simulink model "vel"  (R2022a)
settings: Solver=FixedStepAuto  StartTime=0.0  StopTime=2  FixedStep=1e-3  RelTol=1e-3
undefined symbols (not defined in the file or in its folder): phi, r, theta
libraries: robotlib x12, simulink_extras x8, robotgazebolib x4, slpidlib x1, simulink x1
settings Model: Creator=abiyyumufti  LastModifiedBy=abiyyumufti

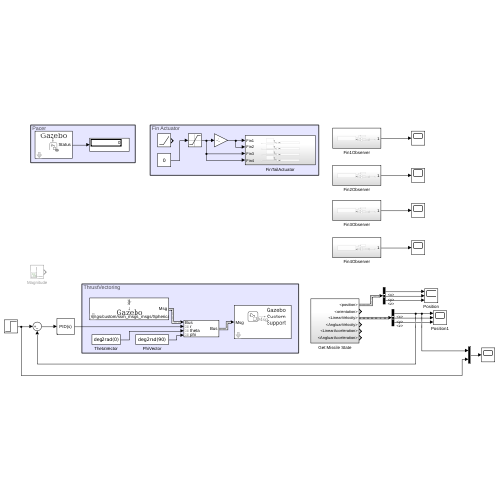
[thumbnail: Simulink's stored preview of the top-level diagram]
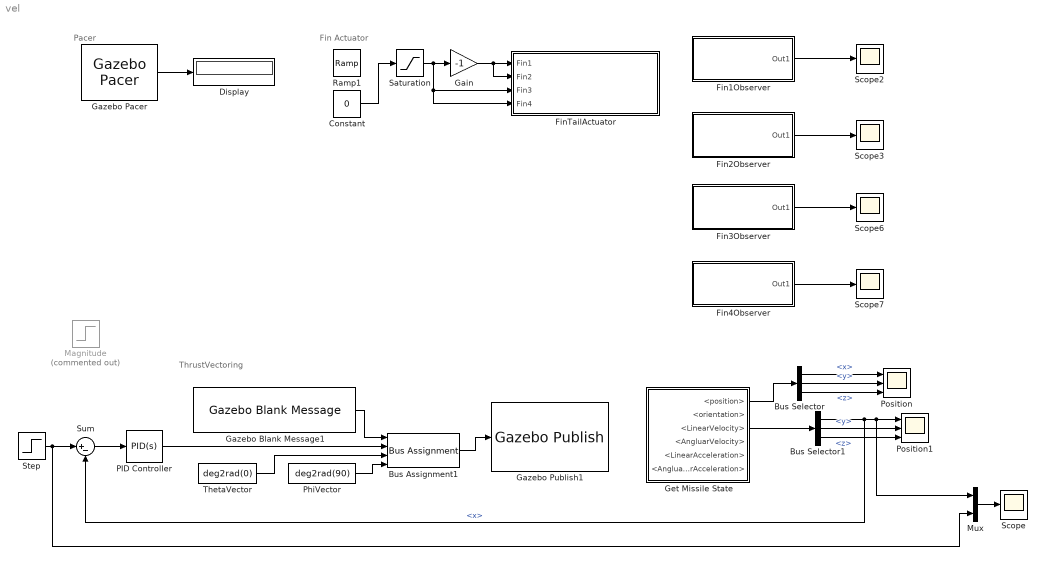
== system vel ==
  note: Fin Actuator
  note: Pacer
  note: ThrustVectoring
  Bus Assignment1 : BusAssignment  AssignedSignals=r,theta,phi
  Bus Selector : BusSelector  OutputSignals=x,y,z
  Bus Selector1 : BusSelector  OutputSignals=x,y,z
  Constant : Constant  Value=0
  Display : Display
  Fin1Observer : Subsystem
  Fin2Observer : Subsystem
  Fin3Observer : Subsystem
  Fin4Observer : Subsystem
  FinTailActuator : Subsystem
  Gain : Gain  Gain=-1
  Gazebo Blank Message1 : robotgazebolib/Gazebo Blank Message  msgType=gazebo_msgs/custom/ssm_msgs_msgs/SphericalVector  sampleTime=0.001  busName='Gazebo_SL_Bus_gazebo_msgs_custom_ssm_msgs_msgs_SphericalVector'
      settings: SourceProductBaseCode=RO
  Gazebo Pacer : robotgazebolib/Gazebo Pacer  ResetBehavior=Reset Gazebo simulation time and scene  SampleTime=0.001
      settings: SourceProductBaseCode=RO
  Gazebo Publish1 : robotgazebolib/Gazebo Publish  topicSource=Specify your own  topic=/gazebo/my_world/thrust_force  messageType=gazebo_msgs/custom/ssm_msgs_msgs/SphericalVector  sampleTime=0.001
      settings: SourceProductBaseCode=RO
  Get Missile State : Subsystem
  Magnitude : Step  Commented=on  Time=2  Before=80000  After=0  SampleTime=0
  Mux : Mux  Inputs=2
  PID Controller : slpidlib/PID Controller  Controller=PID  Form=Parallel  TimeDomain=Continuous-time  UseExternalTs=off  SampleTime=-1  IntegratorMethod=Forward Euler  FilterMethod=Forward Euler  ControllerParametersSource=internal  P=10000  I=0  UseKiTs=off  D=15  N=100  UseFilter=on  TunerSelectOption=Transfer Function Based (PID Tuner App)  InitialConditionSource=internal  InitialConditionForIntegrator=0  InitialConditionForFilter=0  DifferentiatorICPrevScaledInput=0  ExternalReset=none  TrackingMode=off  Kt=1  LimitOutput=off  SatLimitsSource=internal  UpperSaturationLimit=inf  LowerSaturationLimit=-inf  LinearizeAsGain=on  AntiWindupMode=none  Kb=1  POutMin=[]  POutMax=[]  IOutMin=[]  IOutMax=[]  DOutMin=[]  DOutMax=[]  NOutMin=[]  NOutMax=[]  SumOutMin=[]  SumOutMax=[]  SaturationOutMin=[]  SaturationOutMax=[]  PParamMin=[]  PParamMax=[]  IParamMin=[]  IParamMax=[]  DParamMin=[]  DParamMax=[]  NParamMin=[]  NParamMax=[]  KbParamMin=[]  KbParamMax=[]  KtParamMin=[]  KtParamMax=[]  KbOutMin=[]  KbOutMax=[]  KtOutMin=[]  KtOutMax=[]  IntegratorOutMin=[]  IntegratorOutMax=[]  FilterOutMin=[]  FilterOutMax=[]  SumI1OutMin=[]  SumI1OutMax=[]  SumI2OutMin=[]  SumI2OutMax=[]  SumI3OutMin=[]  SumI3OutMax=[]  SumI4OutMin=[]  SumI4OutMax=[]  SumDOutMin=[]  SumDOutMax=[]  DifferentiatorOutMin=[]  DifferentiatorOutMax=[]  FilterDiffOutCoefMin=[]  FilterDiffOutCoefMax=[]  ReciprocalOutMin=[]  ReciprocalOutMax=[]  SumDenOutMin=[]  SumDenOutMax=[]  SumNumOutMin=[]  SumNumOutMax=[]  DivideOutMin=[]  DivideOutMax=[]  UdiffTsProdOutMin=[]  UdiffTsProdOutMax=[]  NTsProdOutMin=[]  NTsProdOutMax=[]  UintegralTsProdOutMin=[]  UintegralTsProdOutMax=[]  UngainTsProdOutMin=[]  UngainTsProdOutMax=[]  IntegratorContinuousStateAttributes=''  IntegratorStateMustResolveToSignalObject=off  IntegratorRTWStateStorageClass=Auto  FilterContinuousStateAttributes=''  FilterStateMustResolveToSignalObject=off  FilterRTWStateStorageClass=Auto  ParallelPVariant=InternalParameters  IdealPVariant=Disabled  IVariant=InternalParameters  DVariant=InternalParameters  IntegratorVariant=Continuous  SatVariant=Disabled  AWVariant=Passthrough  PCopyVariant=Disabled  TRVariant=Disabled  FdbkBlocksVariant=Forward  IdealPFdbkVariant=Disabled  SatFdbkVariant=Disabled  DerivativeFilterVariant=ContFilter  NVariant=InternalParameters  NCopyVariant=Disabled  FilterICVariant=InternalICsFilter  IntegratorICVariant=InternalICs  ExternalResetVariant=Disabled  TRSumVariant=Passthrough  SumFdbkVariant=Disabled  SumVariant=Sum_PID  TsampFilterVariant=InternalTs  TsampNgainVariant=Passthrough  TsampIntegralVariant=Passthrough  ExternalSaturationOutDataTypeStr=Inherit: Same as second input  aMode=0
  PhiVector : Constant  Value=deg2rad(90)
  Position : Scope  NumInputPorts=3
  Position1 : Scope  NumInputPorts=3
  Ramp1 : simulink/Sources/Ramp  slope=deg2rad(20)/2  start=3  InitialOutput=0
  Saturation : Saturate  UpperLimit=deg2rad(10)  LowerLimit=-deg2rad(10)
  Scope{,2..3,6..7} (5 alike) : Scope
  Step : Step  Time=1e-3  After=250  SampleTime=0
  Sum : Sum  Inputs=|+-
  ThetaVector : Constant  Value=deg2rad(0)
  wires:
  Gazebo Pacer/1 -> Display/1
  Fin1Observer/1(Out1) -> Scope2/1
  Fin2Observer/1(Out1) -> Scope3/1
  Fin3Observer/1(Out1) -> Scope6/1
  Fin4Observer/1(Out1) -> Scope7/1
  Gain/1 -> FinTailActuator/2(Fin2), FinTailActuator/1(Fin1)
  Constant/1 -> Saturation/1
  Saturation/1 -> FinTailActuator/4(Fin4), FinTailActuator/3(Fin3), Gain/1
  Bus Assignment1/1 -> Gazebo Publish1/1
  ThetaVector/1 -> Bus Assignment1/3
  Gazebo Blank Message1/1 -> Bus Assignment1/1
  PhiVector/1 -> Bus Assignment1/4
  Get Missile State/1(<position>) -> Bus Selector/1
  Bus Selector/1 -> Position/1  "<x>"
  Bus Selector/2 -> Position/2  "<y>"
  Bus Selector/3 -> Position/3  "<z>"
  Bus Selector1/3 -> Position1/3  "<z>"
  Bus Selector1/2 -> Position1/2  "<y>"
  Bus Selector1/1 -> Sum/2, Mux/1, Position1/1  "<x>"
  Get Missile State/3(<LinearVelocity>) -> Bus Selector1/1
  Step/1 -> Mux/2, Sum/1
  Sum/1 -> PID Controller/1
  PID Controller/1 -> Bus Assignment1/2
  Mux/1 -> Scope/1

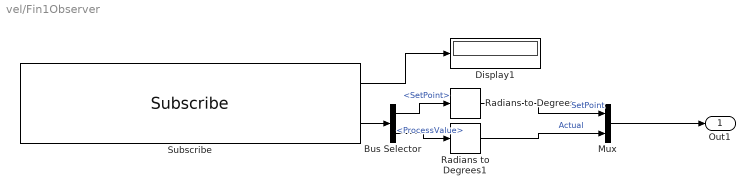
== system vel/Fin1Observer ==
  Bus Selector : BusSelector  OutputSignals=SetPoint,ProcessValue
  Display1 : Display
  Mux : Mux  Inputs=2
  Radians to Degrees : simulink_extras/Transformations/Radians to Degrees
  Radians to Degrees1 : simulink_extras/Transformations/Radians to Degrees
  Subscribe : robotlib/Subscribe  topicSource=Select from ROS network  topic=/model_missile_controller/fins_rev1_position_controller/state  messageType=control_msgs/JointControllerState  SampleTime=-1  legacyBusStruct=off  messageQueueLength=1
  Out1 : Outport
  wires:
  Subscribe/2 -> Bus Selector/1
  Bus Selector/2 -> Radians to Degrees1/1  "<ProcessValue>"
  Subscribe/1 -> Display1/1
  Bus Selector/1 -> Radians to Degrees/1  "<SetPoint>"
  Radians to Degrees1/1 -> Mux/2  "Actual"
  Mux/1 -> Out1/1
  Radians to Degrees/1 -> Mux/1  "SetPoint"

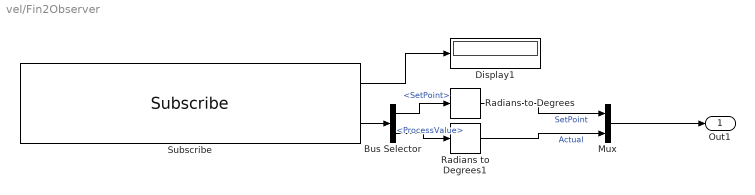
== system vel/Fin2Observer ==
  Bus Selector : BusSelector  OutputSignals=SetPoint,ProcessValue
  Display1 : Display
  Mux : Mux  Inputs=2
  Radians to Degrees : simulink_extras/Transformations/Radians to Degrees
  Radians to Degrees1 : simulink_extras/Transformations/Radians to Degrees
  Subscribe : robotlib/Subscribe  topicSource=Select from ROS network  topic=/model_missile_controller/fins_rev2_position_controller/state  messageType=control_msgs/JointControllerState  SampleTime=-1  legacyBusStruct=off  messageQueueLength=1
  Out1 : Outport
  wires:
  Radians to Degrees/1 -> Mux/1  "SetPoint"
  Mux/1 -> Out1/1
  Radians to Degrees1/1 -> Mux/2  "Actual"
  Bus Selector/1 -> Radians to Degrees/1  "<SetPoint>"
  Subscribe/1 -> Display1/1
  Bus Selector/2 -> Radians to Degrees1/1  "<ProcessValue>"
  Subscribe/2 -> Bus Selector/1

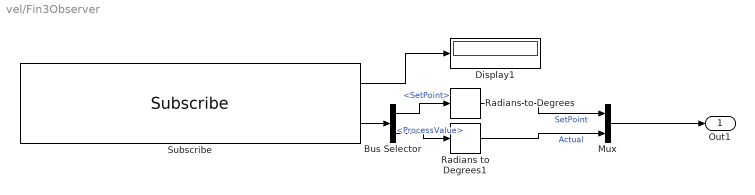
== system vel/Fin3Observer ==
  Bus Selector : BusSelector  OutputSignals=SetPoint,ProcessValue
  Display1 : Display
  Mux : Mux  Inputs=2
  Radians to Degrees : simulink_extras/Transformations/Radians to Degrees
  Radians to Degrees1 : simulink_extras/Transformations/Radians to Degrees
  Subscribe : robotlib/Subscribe  topicSource=Select from ROS network  topic=/model_missile_controller/fins_rev3_position_controller/state  messageType=control_msgs/JointControllerState  SampleTime=-1  legacyBusStruct=off  messageQueueLength=1
  Out1 : Outport
  wires:
  Radians to Degrees/1 -> Mux/1  "SetPoint"
  Mux/1 -> Out1/1
  Radians to Degrees1/1 -> Mux/2  "Actual"
  Bus Selector/1 -> Radians to Degrees/1  "<SetPoint>"
  Subscribe/1 -> Display1/1
  Bus Selector/2 -> Radians to Degrees1/1  "<ProcessValue>"
  Subscribe/2 -> Bus Selector/1

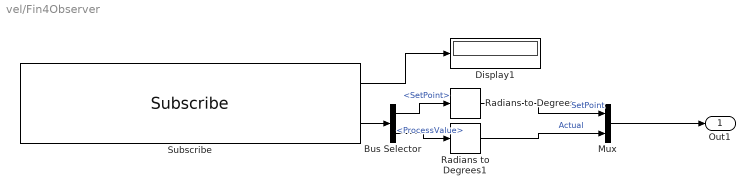
== system vel/Fin4Observer ==
  Bus Selector : BusSelector  OutputSignals=SetPoint,ProcessValue
  Display1 : Display
  Mux : Mux  Inputs=2
  Radians to Degrees : simulink_extras/Transformations/Radians to Degrees
  Radians to Degrees1 : simulink_extras/Transformations/Radians to Degrees
  Subscribe : robotlib/Subscribe  topicSource=Select from ROS network  topic=/model_missile_controller/fins_rev4_position_controller/state  messageType=control_msgs/JointControllerState  SampleTime=-1  legacyBusStruct=off  messageQueueLength=1
  Out1 : Outport
  wires:
  Subscribe/2 -> Bus Selector/1
  Bus Selector/2 -> Radians to Degrees1/1  "<ProcessValue>"
  Subscribe/1 -> Display1/1
  Bus Selector/1 -> Radians to Degrees/1  "<SetPoint>"
  Radians to Degrees1/1 -> Mux/2  "Actual"
  Mux/1 -> Out1/1
  Radians to Degrees/1 -> Mux/1  "SetPoint"

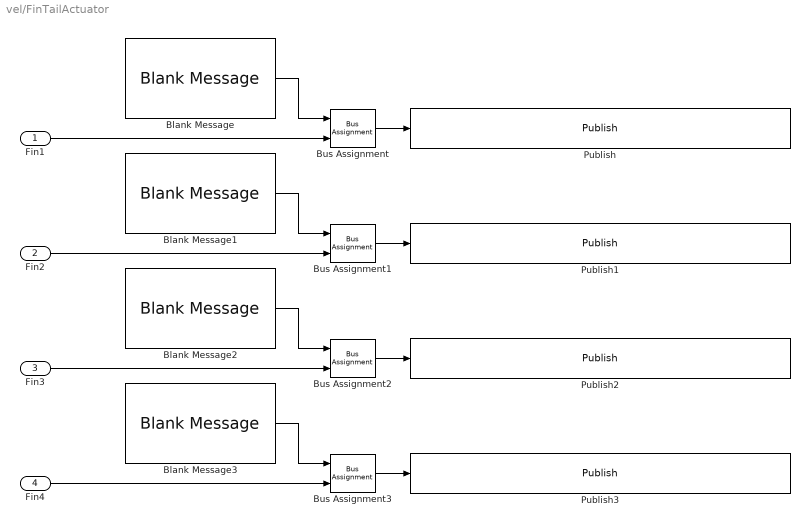
== system vel/FinTailActuator ==
  Fin1 : Inport
  Fin2 : Inport  Port=2
  Fin3 : Inport  Port=3
  Fin4 : Inport  Port=4
  Blank Message{,1..3} (4 alike) : robotlib/Blank Message  messageClass=Message  entityType=std_msgs/Float64  messageType=std_msgs/Float64  SampleTime=inf  legacyBusStruct=off
  Bus Assignment{,1..3} (4 alike) : BusAssignment  AssignedSignals=Data
  Publish : robotlib/Publish  topicSource=Select from ROS network  topic=/model_missile_controller/fins_rev1_position_controller/command  messageType=std_msgs/Float64  legacyBusStruct=off  messageQueueLength=1
  Publish1 : robotlib/Publish  topicSource=Select from ROS network  topic=/model_missile_controller/fins_rev2_position_controller/command  messageType=std_msgs/Float64  legacyBusStruct=off  messageQueueLength=1
  Publish2 : robotlib/Publish  topicSource=Select from ROS network  topic=/model_missile_controller/fins_rev3_position_controller/command  messageType=std_msgs/Float64  legacyBusStruct=off  messageQueueLength=1
  Publish3 : robotlib/Publish  topicSource=Select from ROS network  topic=/model_missile_controller/fins_rev4_position_controller/command  messageType=std_msgs/Float64  legacyBusStruct=off  messageQueueLength=1
  wires:
  Fin1/1 -> Bus Assignment/2
  Bus Assignment3/1 -> Publish3/1
  Blank Message/1 -> Bus Assignment/1
  Fin4/1 -> Bus Assignment3/2
  Bus Assignment1/1 -> Publish1/1
  Blank Message3/1 -> Bus Assignment3/1
  Blank Message2/1 -> Bus Assignment2/1
  Bus Assignment/1 -> Publish/1
  Blank Message1/1 -> Bus Assignment1/1
  Bus Assignment2/1 -> Publish2/1
  Fin2/1 -> Bus Assignment1/2
  Fin3/1 -> Bus Assignment2/2

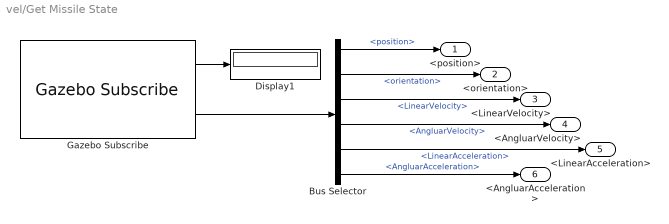
== system vel/Get Missile State ==
  Bus Selector : BusSelector  OutputSignals=Pose.position,Pose.orientation,LinearVelocity,AngluarVelocity,LinearAcceleration,AngluarAcceleration
  Display1 : Display
  Gazebo Subscribe : robotgazebolib/Gazebo Subscribe  topicSource=From Gazebo  topic=/gazebo/my_world/DynamicState  messageType=gazebo_msgs/custom/ssm_msgs_msgs/DynamicState  sampleTime=0.001
      settings: SourceProductBaseCode=RO
  <position> : Outport
  <orientation> : Outport  Port=2
  <LinearVelocity> : Outport  Port=3
  <AngluarVelocity> : Outport  Port=4
  <LinearAcceleration> : Outport  Port=5
  <AngluarAcceleration> : Outport  Port=6
  wires:
  Gazebo Subscribe/2 -> Bus Selector/1
  Gazebo Subscribe/1 -> Display1/1
  Bus Selector/4 -> <AngluarVelocity>/1  "<AngluarVelocity>"
  Bus Selector/6 -> <AngluarAcceleration>/1  "<AngluarAcceleration>"
  Bus Selector/5 -> <LinearAcceleration>/1  "<LinearAcceleration>"
  Bus Selector/1 -> <position>/1  "<position>"
  Bus Selector/3 -> <LinearVelocity>/1  "<LinearVelocity>"
  Bus Selector/2 -> <orientation>/1  "<orientation>"
